simulink model "Ejemplo"  (Simulink 9.3)
settings: Solver=ode3  StartTime=0.0  StopTime=1000  RelTol=1e-3  EnableMultiTasking=on
values from neighbouring files (symbols this model uses):
  Ce0 = 0.543    [TP1.m]
  Ci0 = 1.1367    [TP1.m]
  Fh0 = 0.8946    [TP1.m]
  Fi0 = 1    [TP1.m]
  Th0 = 473    [TP1.m]
  Ti0 = 298    [TP1.m]
undefined symbols (not defined in the file or in its folder): a, b, C0
libraries: simulink_need_slupdate x2
settings Model: Creator=Usuario  LastModifiedBy=Rick Sanchez
settings SolverCC: SolverResetMethod=Robust
settings DebuggingCC: SolverPrmCheckMsg=warning
settings GRTTargetCC: GeneratePreprocessorConditionals=Disable all

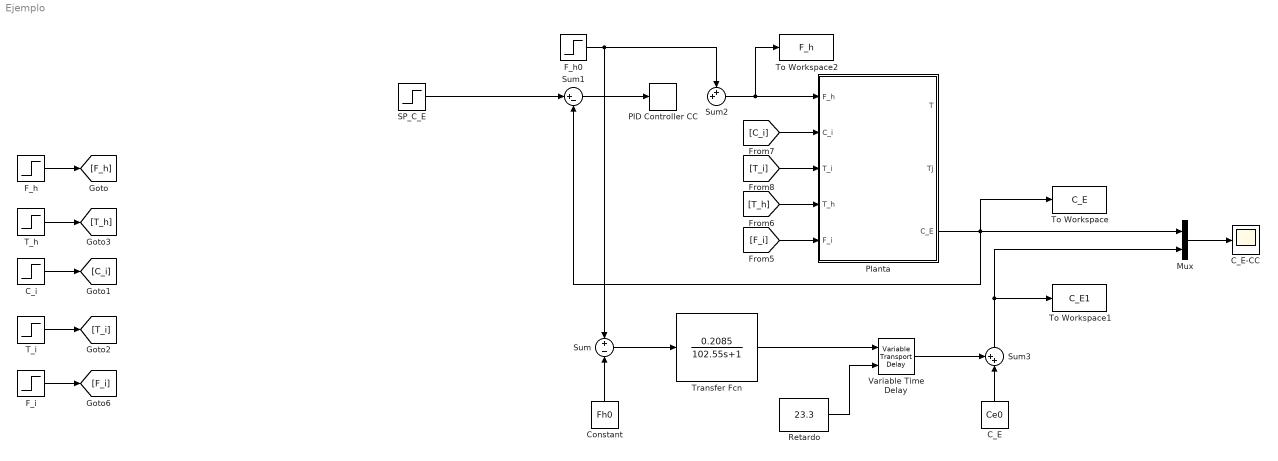
== system Ejemplo ==
  C_E : Constant  Value=Ce0
  C_E-CC : Scope
  C_i : Step  Time=50  Before=Ci0  After=Ci0  SampleTime=1
  Constant : Constant  Value=Fh0
  F_h : Step  Time=83  Before=Fh0  After=Fh0*1  SampleTime=1
  F_h0 : Step  Time=100  Before=Fh0  After=Fh0*1.04  SampleTime=1
  F_i : Step  Time=50  Before=Fi0  After=Fi0  SampleTime=1
  Mux : Mux  Inputs=2
  PID Controller CC : simulink_need_slupdate/PID Controller  P=12.9  I=12.9/52.5  D=12.9*8.1
      settings: SourceProductName=Simulink
  Planta : Subsystem
  Retardo : Constant  Value=23.3
  SP_C_E : Step  Time=100  Before=Ce0  After=Ce0*1.00  SampleTime=0
  Sum : Sum  Inputs=+-
  Sum1 : Sum  Inputs=|+-
  Sum2 : Sum  Inputs=++|
  Sum3 : Sum  Inputs=++|
  T_h : Step  Time=50  Before=Th0  After=Th0  SampleTime=1
  T_i : Step  Time=100  Before=Ti0  After=Ti0*1.00  SampleTime=1
  To Workspace : ToWorkspace  VariableName=C_E
  To Workspace1 : ToWorkspace  VariableName=C_E1
  To Workspace2 : ToWorkspace  VariableName=F_h
  Transfer Fcn : TransferFcn  Numerator=[0.2085]  Denominator=[102.55 1]
  Variable Time Delay : VariableTransportDelay  MaximumDelay=10  TransDelayFeedthrough=on
  wires:
  F_h/1 -> [F_h]
  C_i/1 -> [C_i]
  T_i/1 -> [T_i]
  T_h/1 -> [T_h]
  F_i/1 -> [F_i]
  Sum/1 -> Transfer Fcn/1
  Variable Time Delay/1 -> Sum3/1
  Transfer Fcn/1 -> Variable Time Delay/1
  Sum2/1 -> To Workspace2/1, Planta/1(F_h)
  Constant/1 -> Sum/2
  [C_i] -> Planta/2(C_i)
  [T_i] -> Planta/3(T_i)
  Retardo/1 -> Variable Time Delay/2
  Mux/1 -> C_E-CC/1
  [T_h] -> Planta/4(T_h)
  F_h0/1 -> Sum/1, Sum2/1
  Planta/3(C_E) -> To Workspace/1, Sum1/2, Mux/1
  [F_i] -> Planta/5(F_i)
  SP_C_E/1 -> Sum1/1
  Sum1/1 -> PID Controller CC/1
  C_E/1 -> Sum3/2
  Sum3/1 -> Mux/2, To Workspace1/1

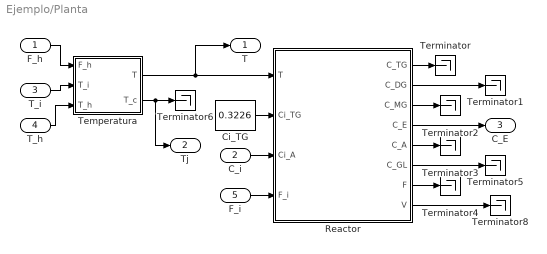
== system Ejemplo/Planta ==
  F_h : Inport
  C_i : Inport  Port=2
  T_i : Inport  Port=3
  T_h : Inport  Port=4
  F_i : Inport  Port=5
  Ci_TG : Constant  Value=0.3226
  Reactor : Subsystem
  Temperatura : Subsystem
  Terminator{,1..6,8} (8 alike) : Terminator
  T : Outport
  Tj : Outport  Port=2
  C_E : Outport  Port=3
  wires:
  Ci_TG/1 -> Reactor/2(Ci_TG)
  F_i/1 -> Reactor/4(F_i)
  Reactor/1(C_TG) -> Terminator/1
  Reactor/2(C_DG) -> Terminator1/1
  Reactor/3(C_MG) -> Terminator2/1
  Reactor/5(C_A) -> Terminator3/1
  Reactor/7(F) -> Terminator4/1
  Reactor/6(C_GL) -> Terminator5/1
  Reactor/8(V) -> Terminator8/1
  Temperatura/2(T_c) -> Terminator6/1, Tj/1
  F_h/1 -> Temperatura/1(F_h)
  Reactor/4(C_E) -> C_E/1
  C_i/1 -> Reactor/3(Ci_A)
  Temperatura/1(T) -> Reactor/1(T), T/1
  T_h/1 -> Temperatura/3(T_h)
  T_i/1 -> Temperatura/2(T_i)

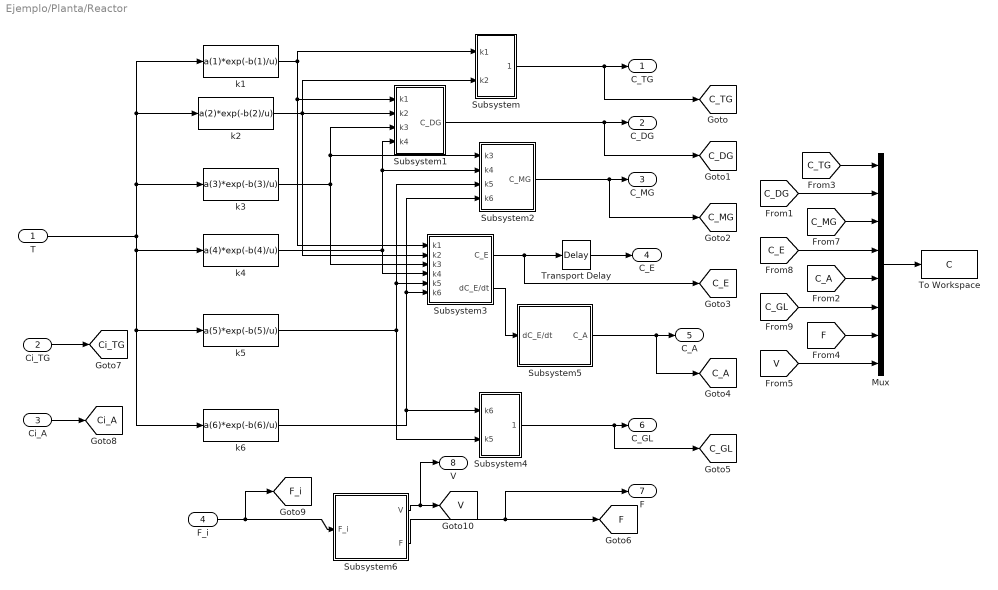
== system Ejemplo/Planta/Reactor ==
  T : Inport
  Ci_TG : Inport  Port=2
  Ci_A : Inport  Port=3
  F_i : Inport  Port=4
  Mux : Mux  Inputs=8
  Subsystem : Subsystem
  Subsystem1 : Subsystem
  Subsystem2 : Subsystem
  Subsystem3 : Subsystem
  Subsystem4 : Subsystem
  Subsystem5 : Subsystem
  Subsystem6 : Subsystem
  To Workspace : ToWorkspace  VariableName=C  SampleTime=-1
  Transport Delay : TransportDelay  DelayTime=10  InitialOutput=C0(4)
  k1 : Fcn  Expr=a(1)*exp(-b(1)/u)
  k2 : Fcn  Expr=a(2)*exp(-b(2)/u)
  k3 : Fcn  Expr=a(3)*exp(-b(3)/u)
  k4 : Fcn  Expr=a(4)*exp(-b(4)/u)
  k5 : Fcn  Expr=a(5)*exp(-b(5)/u)
  k6 : Fcn  Expr=a(6)*exp(-b(6)/u)
  C_TG : Outport
  C_DG : Outport  Port=2
  C_MG : Outport  Port=3
  C_E : Outport  Port=4
  C_A : Outport  Port=5
  C_GL : Outport  Port=6
  F : Outport  Port=7
  V : Outport  Port=8
  tag scope: C_A=global, C_DG=global, C_E=global, C_GL=global, C_MG=global, C_TG=global, Ci_A=global, Ci_TG=global, F=global, F_i=global, V=global
  wires:
  Subsystem4/1(C_GL) -> C_GL/1, [C_GL]
  Subsystem5/1(C_A) -> C_A/1, [C_A]
  Subsystem3/1(C_E) -> [C_E], Transport Delay/1
  Subsystem2/1(C_MG) -> C_MG/1, [C_MG]
  Subsystem1/1(C_DG) -> C_DG/1, [C_DG]
  T/1 -> k4/1, k6/1, k5/1, k1/1, k2/1, k3/1
  k1/1 -> Subsystem/1(k1), Subsystem1/1(k1), Subsystem3/1(k1)
  k2/1 -> Subsystem/2(k2), Subsystem1/2(k2), Subsystem3/2(k2)
  Subsystem/1(C_TG) -> C_TG/1, [C_TG]
  k3/1 -> Subsystem1/3(k3), Subsystem2/1(k3), Subsystem3/3(k3)
  k4/1 -> Subsystem1/4(k4), Subsystem2/2(k4), Subsystem3/4(k4)
  k5/1 -> Subsystem2/3(k5), Subsystem3/5(k5), Subsystem4/2(k5)
  k6/1 -> Subsystem2/4(k6), Subsystem3/6(k6), Subsystem4/1(k6)
  Subsystem3/2(dC_E/dt) -> Subsystem5/1(dC_E/dt)
  Ci_TG/1 -> [Ci_TG]
  Ci_A/1 -> [Ci_A]
  Subsystem6/1(V) -> [V], V/1
  Subsystem6/2(F) -> F/1, [F]
  F_i/1 -> Subsystem6/1(F_i), [F_i]
  Transport Delay/1 -> C_E/1
  [C_TG] -> Mux/1
  [C_DG] -> Mux/2
  [C_MG] -> Mux/3
  [C_E] -> Mux/4
  [C_A] -> Mux/5
  [C_GL] -> Mux/6
  Mux/1 -> To Workspace/1
  [F] -> Mux/7
  [V] -> Mux/8

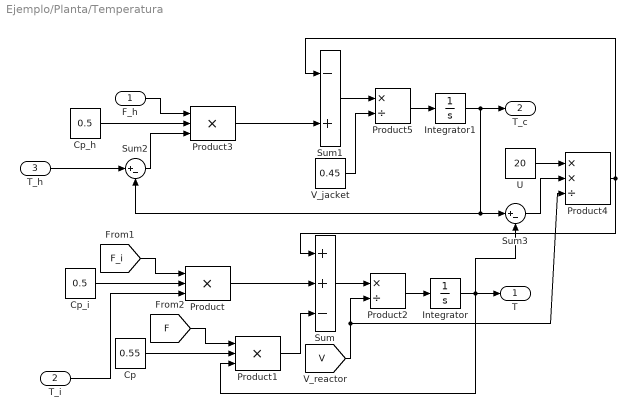
== system Ejemplo/Planta/Temperatura ==
  F_h : Inport
  T_i : Inport  Port=2
  T_h : Inport  Port=3
  Cp : Constant  Value=0.55
  Cp_h : Constant  Value=0.5
  Cp_i : Constant  Value=0.5
  Integrator : Integrator  InitialCondition=323
  Integrator1 : Integrator  InitialCondition=408.95
  Product : Product  Inputs=3  SaturateOnIntegerOverflow=on  RndMeth=Zero  InputSameDT=on  OutDataTypeStr=Inherit: Same as first input
  Product1 : Product  Inputs=3  SaturateOnIntegerOverflow=on  RndMeth=Zero  InputSameDT=on  OutDataTypeStr=Inherit: Same as first input
  Product2 : Product  Inputs=*/  SaturateOnIntegerOverflow=on  RndMeth=Zero  InputSameDT=on  OutDataTypeStr=Inherit: Same as first input
  Product3 : Product  Inputs=3  SaturateOnIntegerOverflow=on  RndMeth=Zero  InputSameDT=on  OutDataTypeStr=Inherit: Same as first input
  Product4 : Product  Inputs=**/  SaturateOnIntegerOverflow=on  RndMeth=Zero  InputSameDT=on  OutDataTypeStr=Inherit: Same as first input
  Product5 : Product  Inputs=*/  SaturateOnIntegerOverflow=on  RndMeth=Zero  InputSameDT=on  OutDataTypeStr=Inherit: Same as first input
  Sum : Sum  Inputs=++-  SaturateOnIntegerOverflow=on  InputSameDT=on  OutDataTypeStr=Inherit: Same as first input
  Sum1 : Sum  Inputs=-+  SaturateOnIntegerOverflow=on  InputSameDT=on  OutDataTypeStr=Inherit: Same as first input
  Sum2 : Sum  Inputs=|+-  SaturateOnIntegerOverflow=on  InputSameDT=on  OutDataTypeStr=Inherit: Same as first input
  Sum3 : Sum  Inputs=|+-  SaturateOnIntegerOverflow=on  InputSameDT=on  OutDataTypeStr=Inherit: Same as first input
  U : Constant  Value=20
  V_jacket : Constant  Value=0.45
  T : Outport
  T_c : Outport  Port=2
  wires:
  Product/1 -> Sum/2
  [F_i] -> Product/1
  Cp_i/1 -> Product/2
  [F] -> Product1/1
  Cp/1 -> Product1/2
  Product1/1 -> Sum/3
  Product2/1 -> Integrator/1
  Sum/1 -> Product2/1
  [V] -> Product2/2, Product4/3
  Integrator/1 -> T/1, Sum3/2, Product1/3
  Product3/1 -> Sum1/2
  F_h/1 -> Product3/1
  Cp_h/1 -> Product3/2
  Sum2/1 -> Product3/3
  Product5/1 -> Integrator1/1
  Sum1/1 -> Product5/1
  V_jacket/1 -> Product5/2
  Integrator1/1 -> T_c/1, Sum2/2, Sum3/1
  T_h/1 -> Sum2/1
  U/1 -> Product4/1
  Sum3/1 -> Product4/2
  Product4/1 -> Sum/1, Sum1/1
  T_i/1 -> Product/3

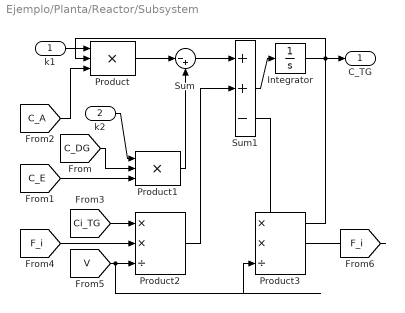
== system Ejemplo/Planta/Reactor/Subsystem ==
  k1 : Inport
  k2 : Inport  Port=2
  Integrator : Integrator  InitialCondition=C0(1)
  Product : Product  Inputs=3  SaturateOnIntegerOverflow=on  RndMeth=Zero  InputSameDT=on  OutDataTypeStr=Inherit: Same as first input
  Product1 : Product  Inputs=3  SaturateOnIntegerOverflow=on  RndMeth=Zero  InputSameDT=on  OutDataTypeStr=Inherit: Same as first input
  Product2 : Product  Inputs=**/  SaturateOnIntegerOverflow=on  RndMeth=Zero  InputSameDT=on  OutDataTypeStr=Inherit: Same as first input
  Product3 : Product  Inputs=**/  SaturateOnIntegerOverflow=on  RndMeth=Zero  InputSameDT=on  OutDataTypeStr=Inherit: Same as first input
  Sum : Sum  Inputs=|-+  SaturateOnIntegerOverflow=on  InputSameDT=on  OutDataTypeStr=Inherit: Same as first input
  Sum1 : Sum  Inputs=++-  SaturateOnIntegerOverflow=on  InputSameDT=on  OutDataTypeStr=Inherit: Same as first input
  C_TG : Outport
  wires:
  Integrator/1 -> Product/2, C_TG/1, Product3/1
  Product/1 -> Sum/1
  Product1/1 -> Sum/2
  [C_DG] -> Product1/2
  [C_E] -> Product1/3
  k1/1 -> Product/1
  k2/1 -> Product1/1
  [C_A] -> Product/3
  Sum1/1 -> Integrator/1
  Sum/1 -> Sum1/1
  [Ci_TG] -> Product2/1
  [F_i] -> Product2/2
  [V] -> Product2/3, Product3/3
  Product2/1 -> Sum1/2
  [F_i] -> Product3/2
  Product3/1 -> Sum1/3

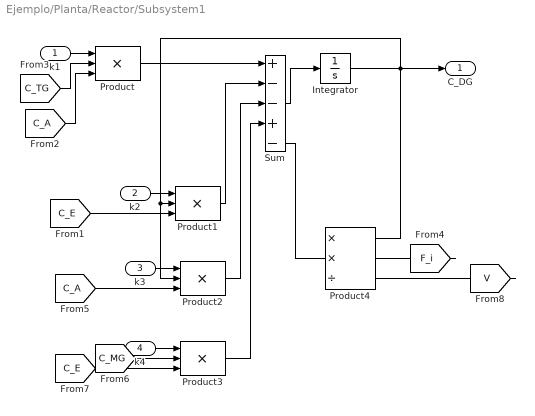
== system Ejemplo/Planta/Reactor/Subsystem1 ==
  k1 : Inport
  k2 : Inport  Port=2
  k3 : Inport  Port=3
  k4 : Inport  Port=4
  Integrator : Integrator  InitialCondition=C0(2)
  Product{,1..3} (4 alike) : Product  Inputs=3  SaturateOnIntegerOverflow=on  RndMeth=Zero  InputSameDT=on  OutDataTypeStr=Inherit: Same as first input
  Product4 : Product  Inputs=**/  SaturateOnIntegerOverflow=on  RndMeth=Zero  InputSameDT=on  OutDataTypeStr=Inherit: Same as first input
  Sum : Sum  Inputs=+--+-  SaturateOnIntegerOverflow=on  InputSameDT=on  OutDataTypeStr=Inherit: Same as first input
  C_DG : Outport
  wires:
  [C_A] -> Product/3
  k2/1 -> Product1/1
  k1/1 -> Product/1
  [C_E] -> Product1/3
  Sum/1 -> Integrator/1
  Product1/1 -> Sum/2
  Product/1 -> Sum/1
  Integrator/1 -> C_DG/1, Product1/2, Product2/2, Product4/1
  [C_TG] -> Product/2
  k3/1 -> Product2/1
  [C_A] -> Product2/3
  k4/1 -> Product3/1
  [C_E] -> Product3/3
  [C_MG] -> Product3/2
  Product2/1 -> Sum/3
  Product3/1 -> Sum/4
  [F_i] -> Product4/2
  Product4/1 -> Sum/5
  [V] -> Product4/3

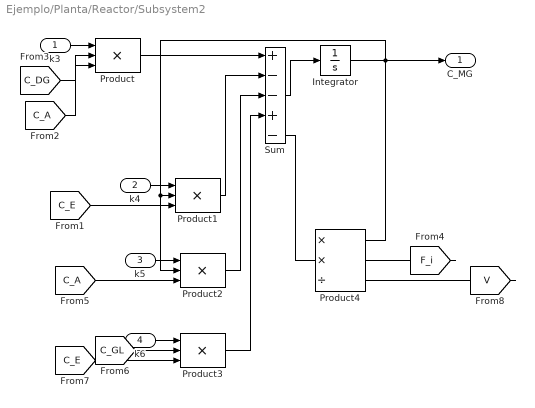
== system Ejemplo/Planta/Reactor/Subsystem2 ==
  k3 : Inport
  k4 : Inport  Port=2
  k5 : Inport  Port=3
  k6 : Inport  Port=4
  Integrator : Integrator  InitialCondition=C0(3)
  Product{,1..3} (4 alike) : Product  Inputs=3  SaturateOnIntegerOverflow=on  RndMeth=Zero  InputSameDT=on  OutDataTypeStr=Inherit: Same as first input
  Product4 : Product  Inputs=**/  SaturateOnIntegerOverflow=on  RndMeth=Zero  InputSameDT=on  OutDataTypeStr=Inherit: Same as first input
  Sum : Sum  Inputs=+--+-  SaturateOnIntegerOverflow=on  InputSameDT=on  OutDataTypeStr=Inherit: Same as first input
  C_MG : Outport
  wires:
  Product3/1 -> Sum/4
  Product2/1 -> Sum/3
  [C_GL] -> Product3/2
  [C_E] -> Product3/3
  k6/1 -> Product3/1
  [C_A] -> Product2/3
  k5/1 -> Product2/1
  [C_DG] -> Product/2
  Integrator/1 -> C_MG/1, Product1/2, Product2/2, Product4/1
  Product/1 -> Sum/1
  Product1/1 -> Sum/2
  Sum/1 -> Integrator/1
  [C_E] -> Product1/3
  k3/1 -> Product/1
  k4/1 -> Product1/1
  [C_A] -> Product/3
  [V] -> Product4/3
  Product4/1 -> Sum/5
  [F_i] -> Product4/2

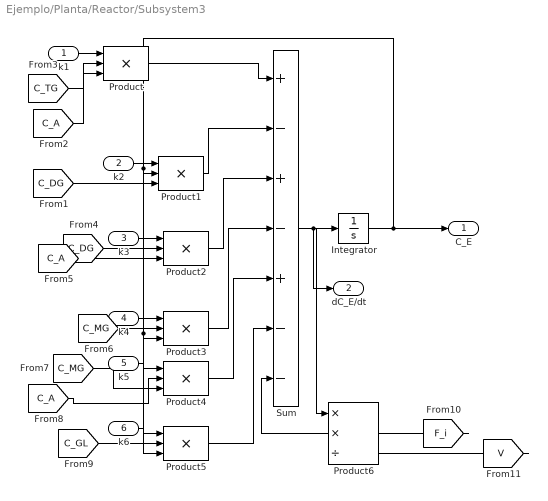
== system Ejemplo/Planta/Reactor/Subsystem3 ==
  k1 : Inport
  k2 : Inport  Port=2
  k3 : Inport  Port=3
  k4 : Inport  Port=4
  k5 : Inport  Port=5
  k6 : Inport  Port=6
  Integrator : Integrator  InitialCondition=C0(4)
  Product{,1..5} (6 alike) : Product  Inputs=3  SaturateOnIntegerOverflow=on  RndMeth=Zero  InputSameDT=on  OutDataTypeStr=Inherit: Same as first input
  Product6 : Product  Inputs=**/  SaturateOnIntegerOverflow=on  RndMeth=Zero  InputSameDT=on  OutDataTypeStr=Inherit: Same as first input
  Sum : Sum  Inputs=+-+-+--  SaturateOnIntegerOverflow=on  InputSameDT=on  OutDataTypeStr=Inherit: Same as first input
  C_E : Outport
  dC_E/dt : Outport  Port=2
  wires:
  [C_A] -> Product/3
  k2/1 -> Product1/1
  k1/1 -> Product/1
  [C_DG] -> Product1/3
  Sum/1 -> Integrator/1, dC_E/dt/1
  Product1/1 -> Sum/2
  Product/1 -> Sum/1
  Integrator/1 -> C_E/1, Product1/2, Product3/3, Product5/3, Product6/1
  [C_TG] -> Product/2
  k3/1 -> Product2/1
  [C_A] -> Product2/3
  k4/1 -> Product3/1
  [C_MG] -> Product3/2
  Product2/1 -> Sum/3
  Product3/1 -> Sum/4
  [C_DG] -> Product2/2
  k5/1 -> Product4/1
  [C_MG] -> Product4/2
  [C_A] -> Product4/3
  Product4/1 -> Sum/5
  k6/1 -> Product5/1
  [C_GL] -> Product5/2
  Product5/1 -> Sum/6
  [V] -> Product6/3
  [F_i] -> Product6/2
  Product6/1 -> Sum/7

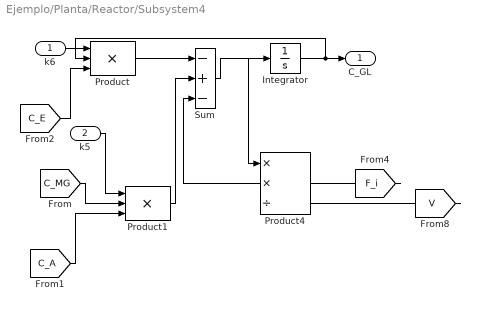
== system Ejemplo/Planta/Reactor/Subsystem4 ==
  k6 : Inport
  k5 : Inport  Port=2
  Integrator : Integrator  InitialCondition=C0(6)
  Product : Product  Inputs=3  SaturateOnIntegerOverflow=on  RndMeth=Zero  InputSameDT=on  OutDataTypeStr=Inherit: Same as first input
  Product1 : Product  Inputs=3  SaturateOnIntegerOverflow=on  RndMeth=Zero  InputSameDT=on  OutDataTypeStr=Inherit: Same as first input
  Product4 : Product  Inputs=**/  SaturateOnIntegerOverflow=on  RndMeth=Zero  InputSameDT=on  OutDataTypeStr=Inherit: Same as first input
  Sum : Sum  Inputs=-+-  SaturateOnIntegerOverflow=on  InputSameDT=on  OutDataTypeStr=Inherit: Same as first input
  C_GL : Outport
  wires:
  [C_E] -> Product/3
  k5/1 -> Product1/1
  k6/1 -> Product/1
  [C_A] -> Product1/3
  [C_MG] -> Product1/2
  Sum/1 -> Integrator/1
  Product1/1 -> Sum/2
  Product/1 -> Sum/1
  Integrator/1 -> C_GL/1, Product/2, Product4/1
  [V] -> Product4/3
  [F_i] -> Product4/2
  Product4/1 -> Sum/3

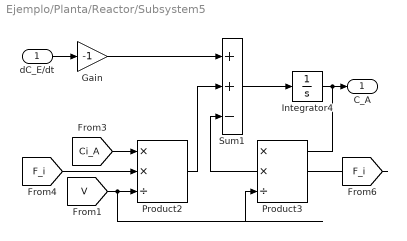
== system Ejemplo/Planta/Reactor/Subsystem5 ==
  dC_E/dt : Inport
  Gain : Gain  Gain=-1  SaturateOnIntegerOverflow=on  OutDataTypeStr=Inherit: Same as input  ParamDataTypeStr=Inherit: Same as input
  Integrator4 : Integrator  InitialCondition=C0(5)
  Product2 : Product  Inputs=**/  SaturateOnIntegerOverflow=on  RndMeth=Zero  InputSameDT=on  OutDataTypeStr=Inherit: Same as first input
  Product3 : Product  Inputs=**/  SaturateOnIntegerOverflow=on  RndMeth=Zero  InputSameDT=on  OutDataTypeStr=Inherit: Same as first input
  Sum1 : Sum  Inputs=++-  SaturateOnIntegerOverflow=on  InputSameDT=on  OutDataTypeStr=Inherit: Same as first input
  C_A : Outport
  wires:
  Integrator4/1 -> C_A/1, Product3/1
  dC_E/dt/1 -> Gain/1
  [Ci_A] -> Product2/1
  [F_i] -> Product2/2
  [V] -> Product2/3, Product3/3
  [F_i] -> Product3/2
  Gain/1 -> Sum1/1
  Sum1/1 -> Integrator4/1
  Product2/1 -> Sum1/2
  Product3/1 -> Sum1/3

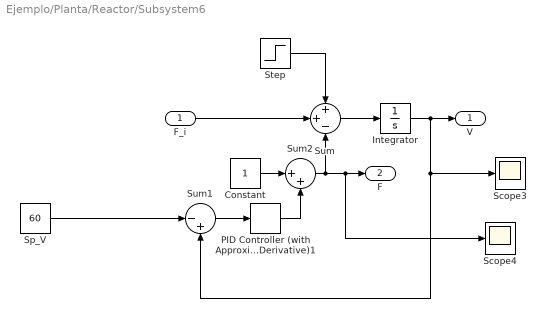
== system Ejemplo/Planta/Reactor/Subsystem6 ==
  F_i : Inport
  Constant : Constant
  Integrator : Integrator  InitialCondition=60
  PID Controller (with Approximate Derivative)1 : simulink_need_slupdate/PID Controller (with Approximate Derivative)  P=2.043  I=1.0215  D=0  N=100
      settings: SourceProductName=Simulink  SourceProductBaseCode=SL
  Scope3 : Scope
  Scope4 : Scope
  Sp_V : Constant  Value=60
  Step : Step  Time=50  After=0  SampleTime=0
  Sum : Sum  Inputs=++-  SaturateOnIntegerOverflow=on  InputSameDT=on  OutDataTypeStr=Inherit: Same as first input
  Sum1 : Sum  Inputs=|-+  SaturateOnIntegerOverflow=on  InputSameDT=on  OutDataTypeStr=Inherit: Same as first input
  Sum2 : Sum  Inputs=|++  SaturateOnIntegerOverflow=on  InputSameDT=on  OutDataTypeStr=Inherit: Same as first input
  V : Outport
  F : Outport  Port=2
  wires:
  Integrator/1 -> V/1, Sum1/2, Scope3/1
  Sum/1 -> Integrator/1
  Sum1/1 -> PID Controller (with Approximate Derivative)1/1
  Constant/1 -> Sum2/1
  Sum2/1 -> F/1, Scope4/1, Sum/3
  Sp_V/1 -> Sum1/1
  F_i/1 -> Sum/2
  Step/1 -> Sum/1
  PID Controller (with Approximate Derivative)1/1 -> Sum2/2
